simulink model "IEEE30_case"  (R2024b)
settings: Solver=FixedStepAuto  StartTime=0  StopTime=5  FixedStep=1e-7  RelTol=1e-3
values from neighbouring files (symbols this model uses):
  GFL_DFIG_7_C_bus = 0.08    [IEEE30_case_parameters.m]
  GFL_DFIG_7_D_mutual = 2.500000e+3    (= 2500)    [IEEE30_case_parameters.m]
  GFL_DFIG_7_f0 = 60    [IEEE30_case_parameters.m]
  GFL_DFIG_7_gPLLi = 3200    [IEEE30_case_parameters.m]
  GFL_DFIG_7_gPLLp = 650    [IEEE30_case_parameters.m]
  GFL_DFIG_7_H_WT = 0.4    [IEEE30_case_parameters.m]
  GFL_DFIG_7_Hg = 0.8    [IEEE30_case_parameters.m]
  GFL_DFIG_7_Igq_ref = 0    [IEEE30_case_parameters.m]
  GFL_DFIG_7_Ird_ref = 704.45696    [IEEE30_case_parameters.m]
  GFL_DFIG_7_KI_V = -300000    [IEEE30_case_parameters.m]
  GFL_DFIG_7_KP_V = -1000    [IEEE30_case_parameters.m]
  GFL_DFIG_7_Ksh = 1.254300e+4    (= 12543)    [IEEE30_case_parameters.m]
  GFL_DFIG_7_Lg = 0.000483    [IEEE30_case_parameters.m]
  GFL_DFIG_7_Lm_pu = 4    [IEEE30_case_parameters.m]
  GFL_DFIG_7_N = 100    [IEEE30_case_parameters.m]
  GFL_DFIG_7_p = 2    [IEEE30_case_parameters.m]
  GFL_DFIG_7_Pitch = 0    [IEEE30_case_parameters.m]
  GFL_DFIG_7_R = 44    [IEEE30_case_parameters.m]
  GFL_DFIG_7_Rg = 2.000000e-5    (= 2e-05)    [IEEE30_case_parameters.m]
  GFL_DFIG_7_rho = 1.225    [IEEE30_case_parameters.m]
  GFL_DFIG_7_rPLLi = 4500    [IEEE30_case_parameters.m]
  GFL_DFIG_7_rPLLp = 620    [IEEE30_case_parameters.m]
  GFL_DFIG_7_Rs_pu = 0.011    [IEEE30_case_parameters.m]
  GFL_DFIG_7_Sbase = 2.000000e+6    (= 2000000)    [IEEE30_case_parameters.m]
  GFL_DFIG_7_ugq_ref = 0    [IEEE30_case_parameters.m]
  GFL_DFIG_7_usd_ref = 0    [IEEE30_case_parameters.m]
  GFL_DFIG_7_Vbase = 690    [IEEE30_case_parameters.m]
  GFL_DFIG_7_Vdc_ref = 1200    [IEEE30_case_parameters.m]
  GFL_DFIG_7_wind = 12    [IEEE30_case_parameters.m]
  GFL_DFIG_7_wm_ref = 518.184209    [IEEE30_case_parameters.m]
  SG_D_13_D = 0.01056    [IEEE30_case_parameters.m]
  SG_D_13_EnableSaturation = 0    [IEEE30_case_parameters.m]
  SG_D_13_f0 = 60    [IEEE30_case_parameters.m]
  SG_D_13_H = 7.5    [IEEE30_case_parameters.m]
  SG_D_13_K_A = 20    [IEEE30_case_parameters.m]
  SG_D_13_K_E = 1.000000e+1    (= 10)    [IEEE30_case_parameters.m]
  SG_D_13_K_F = 2.363    [IEEE30_case_parameters.m]
  SG_D_13_K_s = 0.5    [IEEE30_case_parameters.m]
  SG_D_13_R_a = 0.001088    [IEEE30_case_parameters.m]
  SG_D_13_S_A = 1    [IEEE30_case_parameters.m]
  SG_D_13_S_B = 0.103    [IEEE30_case_parameters.m]
  SG_D_13_S_N = 10.659857    [IEEE30_case_parameters.m]
  SG_D_13_SpeedPara = 200    [IEEE30_case_parameters.m]
  SG_D_13_T_0 = 0.370163    [IEEE30_case_parameters.m]
  SG_D_13_T_1 = 0.3    [IEEE30_case_parameters.m]
  SG_D_13_T_2 = 0.05    [IEEE30_case_parameters.m]
  SG_D_13_T_3 = 0.02    [IEEE30_case_parameters.m]
  SG_D_13_T_4 = 0.005    [IEEE30_case_parameters.m]
  SG_D_13_T_A = 0.02    [IEEE30_case_parameters.m]
  SG_D_13_T_dd = 8.000000e+0    (= 8)    [IEEE30_case_parameters.m]
  SG_D_13_T_ddd = 0.04    [IEEE30_case_parameters.m]
  SG_D_13_T_E = 0.314    [IEEE30_case_parameters.m]
  SG_D_13_T_F = 0.35    [IEEE30_case_parameters.m]
  SG_D_13_T_qd = 0.8    [IEEE30_case_parameters.m]
  SG_D_13_T_qdd = 0.02    [IEEE30_case_parameters.m]
  SG_D_13_T_speed = 0.1    [IEEE30_case_parameters.m]
  SG_D_13_T_w = 0.5    [IEEE30_case_parameters.m]
  SG_D_13_V_ref = 1.696619    [IEEE30_case_parameters.m]
  SG_D_13_w_ref = 376.991118    [IEEE30_case_parameters.m]
  SG_D_13_x_d = 1.9    [IEEE30_case_parameters.m]
  SG_D_13_x_dd = 0.302    [IEEE30_case_parameters.m]
  SG_D_13_x_ddd = 0.204    [IEEE30_case_parameters.m]
  SG_D_13_x_l = 0.05    [IEEE30_case_parameters.m]
  SG_D_13_x_q = 1.3    [IEEE30_case_parameters.m]
  SG_D_13_x_qd = 0.5    [IEEE30_case_parameters.m]
  SG_D_13_x_qdd = 0.3    [IEEE30_case_parameters.m]
  SG_D_1_D = 0.01056    [IEEE30_case_parameters.m]
  SG_D_1_EnableSaturation = 0    [IEEE30_case_parameters.m]
  SG_D_1_f0 = 60    [IEEE30_case_parameters.m]
  SG_D_1_H = 7.5    [IEEE30_case_parameters.m]
  SG_D_1_K_A = 20    [IEEE30_case_parameters.m]
  SG_D_1_K_E = 1.000000e+1    (= 10)    [IEEE30_case_parameters.m]
  SG_D_1_K_F = 2.363    [IEEE30_case_parameters.m]
  SG_D_1_K_s = 0.5    [IEEE30_case_parameters.m]
  SG_D_1_R_a = 0.001088    [IEEE30_case_parameters.m]
  SG_D_1_S_A = 1    [IEEE30_case_parameters.m]
  SG_D_1_S_B = 0.103    [IEEE30_case_parameters.m]
  SG_D_1_S_N = 10.659857    [IEEE30_case_parameters.m]
  SG_D_1_SpeedPara = 200    [IEEE30_case_parameters.m]
  SG_D_1_T_0 = 0.259812    [IEEE30_case_parameters.m]
  SG_D_1_T_1 = 0.3    [IEEE30_case_parameters.m]
  SG_D_1_T_2 = 0.05    [IEEE30_case_parameters.m]
  SG_D_1_T_3 = 0.02    [IEEE30_case_parameters.m]
  SG_D_1_T_4 = 0.005    [IEEE30_case_parameters.m]
  SG_D_1_T_A = 0.02    [IEEE30_case_parameters.m]
  SG_D_1_T_dd = 8.000000e+0    (= 8)    [IEEE30_case_parameters.m]
  SG_D_1_T_ddd = 0.04    [IEEE30_case_parameters.m]
  SG_D_1_T_E = 0.314    [IEEE30_case_parameters.m]
  SG_D_1_T_F = 0.35    [IEEE30_case_parameters.m]
  SG_D_1_T_qd = 0.8    [IEEE30_case_parameters.m]
  SG_D_1_T_qdd = 0.02    [IEEE30_case_parameters.m]
  SG_D_1_T_speed = 0.1    [IEEE30_case_parameters.m]
  SG_D_1_T_w = 0.5    [IEEE30_case_parameters.m]
  SG_D_1_V_ref = 1.544107    [IEEE30_case_parameters.m]
  SG_D_1_w_ref = 376.991118    [IEEE30_case_parameters.m]
  SG_D_1_x_d = 1.9    [IEEE30_case_parameters.m]
  SG_D_1_x_dd = 0.302    [IEEE30_case_parameters.m]
  SG_D_1_x_ddd = 0.204    [IEEE30_case_parameters.m]
  SG_D_1_x_l = 0.05    [IEEE30_case_parameters.m]
  SG_D_1_x_q = 1.3    [IEEE30_case_parameters.m]
  SG_D_1_x_qd = 0.5    [IEEE30_case_parameters.m]
  SG_D_1_x_qdd = 0.3    [IEEE30_case_parameters.m]
  SG_D_22_D = 0.01056    [IEEE30_case_parameters.m]
  SG_D_22_EnableSaturation = 0    [IEEE30_case_parameters.m]
  SG_D_22_f0 = 60    [IEEE30_case_parameters.m]
  SG_D_22_H = 7.5    [IEEE30_case_parameters.m]
  SG_D_22_K_A = 20    [IEEE30_case_parameters.m]
  SG_D_22_K_E = 1.000000e+1    (= 10)    [IEEE30_case_parameters.m]
  SG_D_22_K_F = 2.363    [IEEE30_case_parameters.m]
  SG_D_22_K_s = 0.5    [IEEE30_case_parameters.m]
  SG_D_22_R_a = 0.001088    [IEEE30_case_parameters.m]
  SG_D_22_S_A = 1    [IEEE30_case_parameters.m]
  SG_D_22_S_B = 0.103    [IEEE30_case_parameters.m]
  SG_D_22_S_N = 10.659857    [IEEE30_case_parameters.m]
  SG_D_22_SpeedPara = 200    [IEEE30_case_parameters.m]
  SG_D_22_T_0 = 0.216121    [IEEE30_case_parameters.m]
  SG_D_22_T_1 = 0.3    [IEEE30_case_parameters.m]
  SG_D_22_T_2 = 0.05    [IEEE30_case_parameters.m]
  SG_D_22_T_3 = 0.02    [IEEE30_case_parameters.m]
  SG_D_22_T_4 = 0.005    [IEEE30_case_parameters.m]
  ... (+126 more)
(part 7 of 27)

== system IEEE30_case/AC_1/d_iq_line_10_21_block ==
  note: d_iq_line_10_21 in IEEE30_case
      | $5385.58740615393\,\mathrm{vq}_{\mathrm{bus},10}-161.567622184618\,\mathrm{iq}_{\mathrm{line},10,21}-376.991118430775\,\mathrm{id}_{\mathrm{line},10,21}-5385.58740615393\,\mathrm{vq}_{\mathrm{bus},21}$
      | Automatically generated on 2025-11-01 18:41:58 .
  State_id_line_10_21_eaa10 : Inport
  State_iq_line_10_21_3e3dc : Inport  Port=2
  State_vq_bus_10_d2e20 : Inport  Port=3
  State_vq_bus_21_091f2 : Inport  Port=4
  Add_26c65 : Sum
  Constant_-376.991118430775_c6985 : Constant  Value=-376.991118430775
  Constant_161.567622184618_102ba : Constant  Value=161.567622184618
  Constant_5385.58740615393_07e60 : Constant  Value=5385.58740615393
  Constant_5385.58740615393_39994 : Constant  Value=5385.58740615393
  Product_149d6 : Product
  Product_44b69 : Product
  Product_4a08d : Product
  Product_e31d5 : Product
  Subtract_26c55 : Sum  Inputs=+-
  Subtract_2b805 : Sum  Inputs=+-
  Blockout_d_iq_line_10_21_9f8c0 : Outport
  wires:
  Constant_-376.991118430775_c6985/1 -> Product_44b69/1
  Product_44b69/1 -> Subtract_2b805/1
  State_id_line_10_21_eaa10/1 -> Product_44b69/2
  Constant_161.567622184618_102ba/1 -> Product_149d6/1
  State_iq_line_10_21_3e3dc/1 -> Product_149d6/2
  Product_149d6/1 -> Subtract_2b805/2
  State_vq_bus_10_d2e20/1 -> Product_e31d5/2
  Product_e31d5/1 -> Add_26c65/2
  Constant_5385.58740615393_07e60/1 -> Product_e31d5/1
  Subtract_2b805/1 -> Add_26c65/1
  Product_4a08d/1 -> Subtract_26c55/2
  Constant_5385.58740615393_39994/1 -> Product_4a08d/1
  State_vq_bus_21_091f2/1 -> Product_4a08d/2
  Add_26c65/1 -> Subtract_26c55/1
  Subtract_26c55/1 -> Blockout_d_iq_line_10_21_9f8c0/1

== system IEEE30_case/AC_1/d_iq_line_10_22_block ==
  note: d_iq_line_10_22 in IEEE30_case
      | $2513.27412287183\,\mathrm{vq}_{\mathrm{bus},10}-175.929188601028\,\mathrm{iq}_{\mathrm{line},10,22}-376.991118430775\,\mathrm{id}_{\mathrm{line},10,22}-2513.27412287183\,\mathrm{vq}_{\mathrm{bus},22}$
      | Automatically generated on 2025-11-01 18:42:00 .
  State_id_line_10_22_084f6 : Inport
  State_iq_line_10_22_3080a : Inport  Port=2
  State_vq_bus_10_6b45e : Inport  Port=3
  State_vq_bus_22_cc06f : Inport  Port=4
  Add_09135 : Sum
  Constant_-376.991118430775_75af6 : Constant  Value=-376.991118430775
  Constant_175.929188601028_09936 : Constant  Value=175.929188601028
  Constant_2513.27412287183_cbdf1 : Constant  Value=2513.27412287183
  Constant_2513.27412287183_d3008 : Constant  Value=2513.27412287183
  Product_19b88 : Product
  Product_591c9 : Product
  Product_bc67e : Product
  Product_ee7ea : Product
  Subtract_086ed : Sum  Inputs=+-
  Subtract_aa73f : Sum  Inputs=+-
  Blockout_d_iq_line_10_22_034e5 : Outport
  wires:
  Constant_-376.991118430775_75af6/1 -> Product_ee7ea/1
  State_id_line_10_22_084f6/1 -> Product_ee7ea/2
  Constant_175.929188601028_09936/1 -> Product_19b88/1
  Product_19b88/1 -> Subtract_aa73f/2
  Product_591c9/1 -> Add_09135/2
  Constant_2513.27412287183_cbdf1/1 -> Product_591c9/1
  State_iq_line_10_22_3080a/1 -> Product_19b88/2
  Product_ee7ea/1 -> Subtract_aa73f/1
  State_vq_bus_10_6b45e/1 -> Product_591c9/2
  Subtract_aa73f/1 -> Add_09135/1
  Product_bc67e/1 -> Subtract_086ed/2
  Constant_2513.27412287183_d3008/1 -> Product_bc67e/1
  State_vq_bus_22_cc06f/1 -> Product_bc67e/2
  Add_09135/1 -> Subtract_086ed/1
  Subtract_086ed/1 -> Blockout_d_iq_line_10_22_034e5/1

== system IEEE30_case/AC_1/d_iq_line_12_13_block ==
  note: d_iq_line_12_13 in IEEE30_case
      | $2692.79370307697\,\mathrm{vq}_{\mathrm{bus},12}-376.991118430775\,\mathrm{id}_{\mathrm{line},12,13}-2692.79370307697\,\mathrm{vq}_{\mathrm{bus},13}$
      | Automatically generated on 2025-11-01 18:41:32 .
  State_id_line_12_13_e0b57 : Inport
  State_vq_bus_12_22143 : Inport  Port=2
  State_vq_bus_13_c3943 : Inport  Port=3
  Add_03ba8 : Sum
  Constant_-376.991118430775_53004 : Constant  Value=-376.991118430775
  Constant_2692.79370307697_acbc8 : Constant  Value=2692.79370307697
  Constant_2692.79370307697_b6261 : Constant  Value=2692.79370307697
  Product_60502 : Product
  Product_6a791 : Product
  Product_984e4 : Product
  Subtract_25f30 : Sum  Inputs=+-
  Blockout_d_iq_line_12_13_55f5a : Outport
  wires:
  Constant_-376.991118430775_53004/1 -> Product_6a791/1
  Constant_2692.79370307697_acbc8/1 -> Product_984e4/1
  Product_984e4/1 -> Add_03ba8/2
  Product_6a791/1 -> Add_03ba8/1
  State_id_line_12_13_e0b57/1 -> Product_6a791/2
  Product_60502/1 -> Subtract_25f30/2
  Constant_2692.79370307697_b6261/1 -> Product_60502/1
  State_vq_bus_12_22143/1 -> Product_984e4/2
  State_vq_bus_13_c3943/1 -> Product_60502/2
  Add_03ba8/1 -> Subtract_25f30/1
  Subtract_25f30/1 -> Blockout_d_iq_line_12_13_55f5a/1

== system IEEE30_case/AC_1/d_iq_line_12_14_block ==
  note: d_iq_line_12_14 in IEEE30_case
      | $1449.96584011837\,\mathrm{vq}_{\mathrm{bus},12}-173.995900814204\,\mathrm{iq}_{\mathrm{line},12,14}-376.991118430775\,\mathrm{id}_{\mathrm{line},12,14}-1449.96584011837\,\mathrm{vq}_{\mathrm{bus},14}$
      | Automatically generated on 2025-11-01 18:41:34 .
  State_id_line_12_14_b6e48 : Inport
  State_iq_line_12_14_89ecd : Inport  Port=2
  State_vq_bus_12_dcaec : Inport  Port=3
  State_vq_bus_14_44cc5 : Inport  Port=4
  Add_8fe1c : Sum
  Constant_-376.991118430775_6f91c : Constant  Value=-376.991118430775
  Constant_1449.96584011837_34179 : Constant  Value=1449.96584011837
  Constant_1449.96584011837_b6100 : Constant  Value=1449.96584011837
  Constant_173.995900814204_1440a : Constant  Value=173.995900814204
  Product_07a6c : Product
  Product_0c37e : Product
  Product_14585 : Product
  Product_d0fc4 : Product
  Subtract_a883b : Sum  Inputs=+-
  Subtract_dbef5 : Sum  Inputs=+-
  Blockout_d_iq_line_12_14_a9efb : Outport
  wires:
  State_iq_line_12_14_89ecd/1 -> Product_07a6c/2
  Constant_-376.991118430775_6f91c/1 -> Product_d0fc4/1
  Constant_173.995900814204_1440a/1 -> Product_07a6c/1
  Product_07a6c/1 -> Subtract_dbef5/2
  State_id_line_12_14_b6e48/1 -> Product_d0fc4/2
  Product_d0fc4/1 -> Subtract_dbef5/1
  Constant_1449.96584011837_b6100/1 -> Product_0c37e/1
  State_vq_bus_12_dcaec/1 -> Product_0c37e/2
  Subtract_dbef5/1 -> Add_8fe1c/1
  Product_0c37e/1 -> Add_8fe1c/2
  Product_14585/1 -> Subtract_a883b/2
  Constant_1449.96584011837_34179/1 -> Product_14585/1
  State_vq_bus_14_44cc5/1 -> Product_14585/2
  Add_8fe1c/1 -> Subtract_a883b/1
  Subtract_a883b/1 -> Blockout_d_iq_line_12_14_a9efb/1

== system IEEE30_case/AC_1/d_iq_line_12_15_block ==
  note: d_iq_line_12_15 in IEEE30_case
      | $2899.93168023673\,\mathrm{vq}_{\mathrm{bus},12}-202.995217616571\,\mathrm{iq}_{\mathrm{line},12,15}-376.991118430775\,\mathrm{id}_{\mathrm{line},12,15}-2899.93168023673\,\mathrm{vq}_{\mathrm{bus},15}$
      | Automatically generated on 2025-11-01 18:41:37 .
  State_id_line_12_15_beed2 : Inport
  State_iq_line_12_15_4b1af : Inport  Port=2
  State_vq_bus_12_5723c : Inport  Port=3
  State_vq_bus_15_811f3 : Inport  Port=4
  Add_8ef8f : Sum
  Constant_-376.991118430775_4e1e9 : Constant  Value=-376.991118430775
  Constant_202.995217616571_fe4cc : Constant  Value=202.995217616571
  Constant_2899.93168023673_6dafa : Constant  Value=2899.93168023673
  Constant_2899.93168023673_db74e : Constant  Value=2899.93168023673
  Product_1019c : Product
  Product_410ea : Product
  Product_7c07b : Product
  Product_c4a2c : Product
  Subtract_52a59 : Sum  Inputs=+-
  Subtract_a4dad : Sum  Inputs=+-
  Blockout_d_iq_line_12_15_872fa : Outport
  wires:
  Constant_-376.991118430775_4e1e9/1 -> Product_1019c/1
  Product_1019c/1 -> Subtract_52a59/1
  State_id_line_12_15_beed2/1 -> Product_1019c/2
  Constant_202.995217616571_fe4cc/1 -> Product_410ea/1
  Product_410ea/1 -> Subtract_52a59/2
  State_iq_line_12_15_4b1af/1 -> Product_410ea/2
  Product_7c07b/1 -> Add_8ef8f/2
  Constant_2899.93168023673_6dafa/1 -> Product_7c07b/1
  State_vq_bus_12_5723c/1 -> Product_7c07b/2
  Subtract_52a59/1 -> Add_8ef8f/1
  Constant_2899.93168023673_db74e/1 -> Product_c4a2c/1
  State_vq_bus_15_811f3/1 -> Product_c4a2c/2
  Add_8ef8f/1 -> Subtract_a4dad/1
  Product_c4a2c/1 -> Subtract_a4dad/2
  Subtract_a4dad/1 -> Blockout_d_iq_line_12_15_872fa/1

== system IEEE30_case/AC_1/d_iq_line_12_16_block ==
  note: d_iq_line_12_16 in IEEE30_case
      | $1884.95559215388\,\mathrm{vq}_{\mathrm{bus},12}-169.646003293849\,\mathrm{iq}_{\mathrm{line},12,16}-376.991118430775\,\mathrm{id}_{\mathrm{line},12,16}-1884.95559215388\,\mathrm{vq}_{\mathrm{bus},16}$
      | Automatically generated on 2025-11-01 18:41:39 .
  State_id_line_12_16_32f87 : Inport
  State_iq_line_12_16_057ef : Inport  Port=2
  State_vq_bus_12_19670 : Inport  Port=3
  State_vq_bus_16_185e6 : Inport  Port=4
  Add_44e5e : Sum
  Constant_-376.991118430775_e69c0 : Constant  Value=-376.991118430775
  Constant_169.646003293849_5d481 : Constant  Value=169.646003293849
  Constant_1884.95559215388_470b5 : Constant  Value=1884.95559215388
  Constant_1884.95559215388_79483 : Constant  Value=1884.95559215388
  Product_1478d : Product
  Product_64d0b : Product
  Product_809b3 : Product
  Product_e344e : Product
  Subtract_a6d27 : Sum  Inputs=+-
  Subtract_c23ff : Sum  Inputs=+-
  Blockout_d_iq_line_12_16_07cfb : Outport
  wires:
  Constant_-376.991118430775_e69c0/1 -> Product_64d0b/1
  Product_e344e/1 -> Subtract_c23ff/2
  Product_64d0b/1 -> Subtract_c23ff/1
  State_id_line_12_16_32f87/1 -> Product_64d0b/2
  Constant_169.646003293849_5d481/1 -> Product_e344e/1
  Product_809b3/1 -> Add_44e5e/2
  Constant_1884.95559215388_470b5/1 -> Product_809b3/1
  State_iq_line_12_16_057ef/1 -> Product_e344e/2
  State_vq_bus_12_19670/1 -> Product_809b3/2
  Subtract_c23ff/1 -> Add_44e5e/1
  Product_1478d/1 -> Subtract_a6d27/2
  Constant_1884.95559215388_79483/1 -> Product_1478d/1
  State_vq_bus_16_185e6/1 -> Product_1478d/2
  Add_44e5e/1 -> Subtract_a6d27/1
  Subtract_a6d27/1 -> Blockout_d_iq_line_12_16_07cfb/1

== system IEEE30_case/AC_1/d_iq_line_14_15_block ==
  note: d_iq_line_14_15 in IEEE30_case
      | $1884.95559215388\,\mathrm{vq}_{\mathrm{bus},14}-414.690230273853\,\mathrm{iq}_{\mathrm{line},14,15}-376.991118430775\,\mathrm{id}_{\mathrm{line},14,15}-1884.95559215388\,\mathrm{vq}_{\mathrm{bus},15}$
      | Automatically generated on 2025-11-01 18:41:42 .
  State_id_line_14_15_7494d : Inport
  State_iq_line_14_15_6bca3 : Inport  Port=2
  State_vq_bus_14_61922 : Inport  Port=3
  State_vq_bus_15_80bf7 : Inport  Port=4
  Add_1b324 : Sum
  Constant_-376.991118430775_071d9 : Constant  Value=-376.991118430775
  Constant_1884.95559215388_19c19 : Constant  Value=1884.95559215388
  Constant_1884.95559215388_3b58e : Constant  Value=1884.95559215388
  Constant_414.690230273853_bfc7a : Constant  Value=414.690230273853
  Product_525e6 : Product
  Product_5c681 : Product
  Product_e29bf : Product
  Product_e4297 : Product
  Subtract_00799 : Sum  Inputs=+-
  Subtract_f1741 : Sum  Inputs=+-
  Blockout_d_iq_line_14_15_23a62 : Outport
  wires:
  Constant_-376.991118430775_071d9/1 -> Product_e4297/1
  Constant_414.690230273853_bfc7a/1 -> Product_5c681/1
  Product_5c681/1 -> Subtract_00799/2
  State_id_line_14_15_7494d/1 -> Product_e4297/2
  State_iq_line_14_15_6bca3/1 -> Product_5c681/2
  Product_e4297/1 -> Subtract_00799/1
  State_vq_bus_14_61922/1 -> Product_525e6/2
  Product_525e6/1 -> Add_1b324/2
  Constant_1884.95559215388_3b58e/1 -> Product_525e6/1
  Subtract_00799/1 -> Add_1b324/1
  Product_e29bf/1 -> Subtract_f1741/2
  Constant_1884.95559215388_19c19/1 -> Product_e29bf/1
  Add_1b324/1 -> Subtract_f1741/1
  State_vq_bus_15_80bf7/1 -> Product_e29bf/2
  Subtract_f1741/1 -> Blockout_d_iq_line_14_15_23a62/1

== system IEEE30_case/AC_1/d_iq_line_15_18_block ==
  note: d_iq_line_15_18 in IEEE30_case
      | $1713.59599286716\,\mathrm{vq}_{\mathrm{bus},15}-188.495559215388\,\mathrm{iq}_{\mathrm{line},15,18}-376.991118430775\,\mathrm{id}_{\mathrm{line},15,18}-1713.59599286716\,\mathrm{vq}_{\mathrm{bus},18}$
      | Automatically generated on 2025-11-01 18:41:46 .
  State_id_line_15_18_c7b72 : Inport
  State_iq_line_15_18_85966 : Inport  Port=2
  State_vq_bus_15_ceac7 : Inport  Port=3
  State_vq_bus_18_6e5b1 : Inport  Port=4
  Add_a8775 : Sum
  Constant_-376.991118430775_1952d : Constant  Value=-376.991118430775
  Constant_1713.59599286716_867a5 : Constant  Value=1713.59599286716
  Constant_1713.59599286716_e050c : Constant  Value=1713.59599286716
  Constant_188.495559215388_7a49f : Constant  Value=188.495559215388
  Product_51a61 : Product
  Product_be0d8 : Product
  Product_ded70 : Product
  Product_e1c77 : Product
  Subtract_50270 : Sum  Inputs=+-
  Subtract_cf1ed : Sum  Inputs=+-
  Blockout_d_iq_line_15_18_9343c : Outport
  wires:
  Constant_-376.991118430775_1952d/1 -> Product_be0d8/1
  Constant_188.495559215388_7a49f/1 -> Product_e1c77/1
  Product_e1c77/1 -> Subtract_cf1ed/2
  Product_be0d8/1 -> Subtract_cf1ed/1
  State_id_line_15_18_c7b72/1 -> Product_be0d8/2
  Product_51a61/1 -> Add_a8775/2
  Constant_1713.59599286716_e050c/1 -> Product_51a61/1
  State_iq_line_15_18_85966/1 -> Product_e1c77/2
  State_vq_bus_15_ceac7/1 -> Product_51a61/2
  Subtract_cf1ed/1 -> Add_a8775/1
  Constant_1713.59599286716_867a5/1 -> Product_ded70/1
  State_vq_bus_18_6e5b1/1 -> Product_ded70/2
  Add_a8775/1 -> Subtract_50270/1
  Product_ded70/1 -> Subtract_50270/2
  Subtract_50270/1 -> Blockout_d_iq_line_15_18_9343c/1

== system IEEE30_case/AC_1/d_iq_line_15_23_block ==
  note: d_iq_line_15_23 in IEEE30_case
      | $1884.95559215388\,\mathrm{vq}_{\mathrm{bus},15}-188.495559215388\,\mathrm{iq}_{\mathrm{line},15,23}-376.991118430775\,\mathrm{id}_{\mathrm{line},15,23}-1884.95559215388\,\mathrm{vq}_{\mathrm{bus},23}$
      | Automatically generated on 2025-11-01 18:42:05 .
  State_id_line_15_23_e0160 : Inport
  State_iq_line_15_23_ade94 : Inport  Port=2
  State_vq_bus_15_76336 : Inport  Port=3
  State_vq_bus_23_32b73 : Inport  Port=4
  Add_e2306 : Sum
  Constant_-376.991118430775_e195e : Constant  Value=-376.991118430775
  Constant_188.495559215388_43fcb : Constant  Value=188.495559215388
  Constant_1884.95559215388_4e938 : Constant  Value=1884.95559215388
  Constant_1884.95559215388_b35ae : Constant  Value=1884.95559215388
  Product_00db3 : Product
  Product_516e5 : Product
  Product_90be9 : Product
  Product_b8377 : Product
  Subtract_711a0 : Sum  Inputs=+-
  Subtract_e6dfb : Sum  Inputs=+-
  Blockout_d_iq_line_15_23_620f2 : Outport
  wires:
  Constant_-376.991118430775_e195e/1 -> Product_90be9/1
  Product_90be9/1 -> Subtract_e6dfb/1
  Subtract_711a0/1 -> Blockout_d_iq_line_15_23_620f2/1
  State_id_line_15_23_e0160/1 -> Product_90be9/2
  Constant_188.495559215388_43fcb/1 -> Product_516e5/1
  Product_516e5/1 -> Subtract_e6dfb/2
  State_iq_line_15_23_ade94/1 -> Product_516e5/2
  Product_00db3/1 -> Add_e2306/2
  Constant_1884.95559215388_b35ae/1 -> Product_00db3/1
  State_vq_bus_15_76336/1 -> Product_00db3/2
  Subtract_e6dfb/1 -> Add_e2306/1
  Constant_1884.95559215388_4e938/1 -> Product_b8377/1
  State_vq_bus_23_32b73/1 -> Product_b8377/2
  Add_e2306/1 -> Subtract_711a0/1
  Product_b8377/1 -> Subtract_711a0/2

== system IEEE30_case/AC_1/d_iq_line_16_17_block ==
  note: d_iq_line_16_17 in IEEE30_case
      | $1984.16378121461\,\mathrm{vq}_{\mathrm{bus},16}-158.733102497168\,\mathrm{iq}_{\mathrm{line},16,17}-376.991118430775\,\mathrm{id}_{\mathrm{line},16,17}-1984.16378121461\,\mathrm{vq}_{\mathrm{bus},17}$
      | Automatically generated on 2025-11-01 18:41:44 .
  State_id_line_16_17_721a9 : Inport
  State_iq_line_16_17_c5f3c : Inport  Port=2
  State_vq_bus_16_312ae : Inport  Port=3
  State_vq_bus_17_5c6e8 : Inport  Port=4
  Add_ea472 : Sum
  Constant_-376.991118430775_937ec : Constant  Value=-376.991118430775
  Constant_158.733102497168_9c41c : Constant  Value=158.733102497168
  Constant_1984.16378121461_5691c : Constant  Value=1984.16378121461
  Constant_1984.16378121461_d1a9e : Constant  Value=1984.16378121461
  Product_1c0b5 : Product
  Product_32b71 : Product
  Product_382cd : Product
  Product_3fc5f : Product
  Subtract_3f09d : Sum  Inputs=+-
  Subtract_60968 : Sum  Inputs=+-
  Blockout_d_iq_line_16_17_36e2b : Outport
  wires:
  Product_1c0b5/1 -> Subtract_3f09d/1
  Constant_-376.991118430775_937ec/1 -> Product_1c0b5/1
  State_id_line_16_17_721a9/1 -> Product_1c0b5/2
  Constant_158.733102497168_9c41c/1 -> Product_3fc5f/1
  Product_3fc5f/1 -> Subtract_3f09d/2
  State_iq_line_16_17_c5f3c/1 -> Product_3fc5f/2
  Subtract_60968/1 -> Blockout_d_iq_line_16_17_36e2b/1
  Constant_1984.16378121461_5691c/1 -> Product_382cd/1
  State_vq_bus_16_312ae/1 -> Product_382cd/2
  Subtract_3f09d/1 -> Add_ea472/1
  Product_382cd/1 -> Add_ea472/2
  Product_32b71/1 -> Subtract_60968/2
  Constant_1984.16378121461_d1a9e/1 -> Product_32b71/1
  State_vq_bus_17_5c6e8/1 -> Product_32b71/2
  Add_ea472/1 -> Subtract_60968/1

== system IEEE30_case/AC_1/d_iq_line_18_19_block ==
  note: d_iq_line_18_19 in IEEE30_case
      | $2899.93168023673\,\mathrm{vq}_{\mathrm{bus},18}-173.995900814204\,\mathrm{iq}_{\mathrm{line},18,19}-376.991118430775\,\mathrm{id}_{\mathrm{line},18,19}-2899.93168023673\,\mathrm{vq}_{\mathrm{bus},19}$
      | Automatically generated on 2025-11-01 18:41:48 .
  State_id_line_18_19_8f9c3 : Inport
  State_iq_line_18_19_da0b4 : Inport  Port=2
  State_vq_bus_18_f4e53 : Inport  Port=3
  State_vq_bus_19_d8da0 : Inport  Port=4
  Add_013ce : Sum
  Constant_-376.991118430775_7eb58 : Constant  Value=-376.991118430775
  Constant_173.995900814204_e9e37 : Constant  Value=173.995900814204
  Constant_2899.93168023673_04a9c : Constant  Value=2899.93168023673
  Constant_2899.93168023673_0d6a4 : Constant  Value=2899.93168023673
  Product_2881c : Product
  Product_84c05 : Product
  Product_af8cd : Product
  Product_e9970 : Product
  Subtract_158eb : Sum  Inputs=+-
  Subtract_e49c7 : Sum  Inputs=+-
  Blockout_d_iq_line_18_19_0dac2 : Outport
  wires:
  Constant_-376.991118430775_7eb58/1 -> Product_e9970/1
  Product_e9970/1 -> Subtract_158eb/1
  State_id_line_18_19_8f9c3/1 -> Product_e9970/2
  Constant_173.995900814204_e9e37/1 -> Product_2881c/1
  Product_84c05/1 -> Add_013ce/2
  Constant_2899.93168023673_04a9c/1 -> Product_84c05/1
  State_iq_line_18_19_da0b4/1 -> Product_2881c/2
  State_vq_bus_18_f4e53/1 -> Product_84c05/2
  Product_2881c/1 -> Subtract_158eb/2
  Subtract_158eb/1 -> Add_013ce/1
  Product_af8cd/1 -> Subtract_e49c7/2
  Constant_2899.93168023673_0d6a4/1 -> Product_af8cd/1
  State_vq_bus_19_d8da0/1 -> Product_af8cd/2
  Add_013ce/1 -> Subtract_e49c7/1
  Subtract_e49c7/1 -> Blockout_d_iq_line_18_19_0dac2/1

== system IEEE30_case/AC_1/d_iq_line_19_20_block ==
  note: d_iq_line_19_20 in IEEE30_case
      | $5385.58740615393\,\mathrm{vq}_{\mathrm{bus},19}-161.567622184618\,\mathrm{iq}_{\mathrm{line},19,20}-376.991118430775\,\mathrm{id}_{\mathrm{line},19,20}-5385.58740615393\,\mathrm{vq}_{\mathrm{bus},20}$
      | Automatically generated on 2025-11-01 18:41:50 .
  State_id_line_19_20_b531a : Inport
  State_iq_line_19_20_2451d : Inport  Port=2
  State_vq_bus_19_a0dab : Inport  Port=3
  State_vq_bus_20_72c0e : Inport  Port=4
  Add_bef5a : Sum
  Constant_-376.991118430775_a4716 : Constant  Value=-376.991118430775
  Constant_161.567622184618_2b234 : Constant  Value=161.567622184618
  Constant_5385.58740615393_0368b : Constant  Value=5385.58740615393
  Constant_5385.58740615393_91113 : Constant  Value=5385.58740615393
  Product_5eee0 : Product
  Product_83d90 : Product
  Product_85c6d : Product
  Product_f88ed : Product
  Subtract_a0a7d : Sum  Inputs=+-
  Subtract_ee448 : Sum  Inputs=+-
  Blockout_d_iq_line_19_20_abe71 : Outport
  wires:
  Constant_-376.991118430775_a4716/1 -> Product_5eee0/1
  Constant_161.567622184618_2b234/1 -> Product_85c6d/1
  Product_85c6d/1 -> Subtract_a0a7d/2
  State_id_line_19_20_b531a/1 -> Product_5eee0/2
  State_iq_line_19_20_2451d/1 -> Product_85c6d/2
  Product_83d90/1 -> Add_bef5a/2
  Constant_5385.58740615393_0368b/1 -> Product_83d90/1
  Product_5eee0/1 -> Subtract_a0a7d/1
  State_vq_bus_19_a0dab/1 -> Product_83d90/2
  Subtract_a0a7d/1 -> Add_bef5a/1
  Product_f88ed/1 -> Subtract_ee448/2
  Constant_5385.58740615393_91113/1 -> Product_f88ed/1
  State_vq_bus_20_72c0e/1 -> Product_f88ed/2
  Add_bef5a/1 -> Subtract_ee448/1
  Subtract_ee448/1 -> Blockout_d_iq_line_19_20_abe71/1

== system IEEE30_case/AC_1/d_iq_line_1_2_block ==
  note: d_iq_line_1_2 in IEEE30_case
      | $6283.18530717959\,\mathrm{vq}_{\mathrm{bus},1}-125.663706143592\,\mathrm{iq}_{\mathrm{line},1,2}-376.991118430775\,\mathrm{id}_{\mathrm{line},1,2}-6283.18530717959\,\mathrm{vq}_{\mathrm{bus},2}$
      | Automatically generated on 2025-11-01 18:40:58 .
  State_id_line_1_2_bca8d : Inport
  State_iq_line_1_2_62f2c : Inport  Port=2
  State_vq_bus_1_1d692 : Inport  Port=3
  State_vq_bus_2_54dcd : Inport  Port=4
  Add_b2adf : Sum
  Constant_-376.991118430775_ca98e : Constant  Value=-376.991118430775
  Constant_125.663706143592_a8407 : Constant  Value=125.663706143592
  Constant_6283.18530717959_17d64 : Constant  Value=6283.18530717959
  Constant_6283.18530717959_801ca : Constant  Value=6283.18530717959
  Product_34205 : Product
  Product_a0ca5 : Product
  Product_dcbb8 : Product
  Product_df49a : Product
  Subtract_4031b : Sum  Inputs=+-
  Subtract_ffb91 : Sum  Inputs=+-
  Blockout_d_iq_line_1_2_85e11 : Outport
  wires:
  Constant_-376.991118430775_ca98e/1 -> Product_df49a/1
  Product_dcbb8/1 -> Subtract_4031b/2
  Constant_6283.18530717959_17d64/1 -> Product_dcbb8/1
  Product_df49a/1 -> Subtract_ffb91/1
  State_id_line_1_2_bca8d/1 -> Product_df49a/2
  Constant_125.663706143592_a8407/1 -> Product_a0ca5/1
  Product_34205/1 -> Add_b2adf/2
  State_iq_line_1_2_62f2c/1 -> Product_a0ca5/2
  Constant_6283.18530717959_801ca/1 -> Product_34205/1
  Product_a0ca5/1 -> Subtract_ffb91/2
  State_vq_bus_1_1d692/1 -> Product_34205/2
  Subtract_ffb91/1 -> Add_b2adf/1
  State_vq_bus_2_54dcd/1 -> Product_dcbb8/2
  Add_b2adf/1 -> Subtract_4031b/1
  Subtract_4031b/1 -> Blockout_d_iq_line_1_2_85e11/1

== system IEEE30_case/AC_1/d_iq_line_1_3_block ==
  note: d_iq_line_1_3 in IEEE30_case
      | $1984.16378121461\,\mathrm{vq}_{\mathrm{bus},1}-99.2081890607303\,\mathrm{iq}_{\mathrm{line},1,3}-376.991118430775\,\mathrm{id}_{\mathrm{line},1,3}-1984.16378121461\,\mathrm{vq}_{\mathrm{bus},3}$
      | Automatically generated on 2025-11-01 18:41:00 .
  State_id_line_1_3_ae183 : Inport
  State_iq_line_1_3_f4510 : Inport  Port=2
  State_vq_bus_1_564cd : Inport  Port=3
  State_vq_bus_3_23559 : Inport  Port=4
  Add_e4d90 : Sum
  Constant_-376.991118430775_b2df0 : Constant  Value=-376.991118430775
  Constant_1984.16378121461_0937d : Constant  Value=1984.16378121461
  Constant_1984.16378121461_24c35 : Constant  Value=1984.16378121461
  Constant_99.2081890607303_19836 : Constant  Value=99.2081890607303
  Product_19dbd : Product
  Product_63c3f : Product
  Product_dc168 : Product
  Product_f16ee : Product
  Subtract_53029 : Sum  Inputs=+-
  Subtract_82ef4 : Sum  Inputs=+-
  Blockout_d_iq_line_1_3_dab4a : Outport
  wires:
  Constant_-376.991118430775_b2df0/1 -> Product_63c3f/1
  State_id_line_1_3_ae183/1 -> Product_63c3f/2
  Constant_99.2081890607303_19836/1 -> Product_19dbd/1
  Product_19dbd/1 -> Subtract_53029/2
  State_iq_line_1_3_f4510/1 -> Product_19dbd/2
  Product_f16ee/1 -> Add_e4d90/2
  Product_63c3f/1 -> Subtract_53029/1
  Constant_1984.16378121461_0937d/1 -> Product_f16ee/1
  State_vq_bus_1_564cd/1 -> Product_f16ee/2
  Subtract_53029/1 -> Add_e4d90/1
  Product_dc168/1 -> Subtract_82ef4/2
  Constant_1984.16378121461_24c35/1 -> Product_dc168/1
  State_vq_bus_3_23559/1 -> Product_dc168/2
  Add_e4d90/1 -> Subtract_82ef4/1
  Subtract_82ef4/1 -> Blockout_d_iq_line_1_3_dab4a/1

== system IEEE30_case/AC_1/d_iq_line_21_22_block ==
  note: d_iq_line_21_22 in IEEE30_case
      | $18849.5559215388\,\mathrm{vq}_{\mathrm{bus},21}-188.495559215388\,\mathrm{iq}_{\mathrm{line},21,22}-376.991118430775\,\mathrm{id}_{\mathrm{line},21,22}-18849.5559215388\,\mathrm{vq}_{\mathrm{bus},22}$
      | Automatically generated on 2025-11-01 18:42:02 .
  State_id_line_21_22_6fd19 : Inport
  State_iq_line_21_22_2fa40 : Inport  Port=2
  State_vq_bus_21_8118e : Inport  Port=3
  State_vq_bus_22_8ed98 : Inport  Port=4
  Add_1c3f8 : Sum
  Constant_-376.991118430775_126f8 : Constant  Value=-376.991118430775
  Constant_188.495559215388_db26c : Constant  Value=188.495559215388
  Constant_18849.5559215388_0d0d0 : Constant  Value=18849.5559215388
  Constant_18849.5559215388_e3d62 : Constant  Value=18849.5559215388
  Product_03a6b : Product
  Product_08fdc : Product
  Product_209a0 : Product
  Product_6e1ba : Product
  Subtract_39b85 : Sum  Inputs=+-
  Subtract_e1a2e : Sum  Inputs=+-
  Blockout_d_iq_line_21_22_19dd1 : Outport
  wires:
  State_iq_line_21_22_2fa40/1 -> Product_6e1ba/2
  Constant_-376.991118430775_126f8/1 -> Product_03a6b/1
  Constant_188.495559215388_db26c/1 -> Product_6e1ba/1
  Product_6e1ba/1 -> Subtract_39b85/2
  State_id_line_21_22_6fd19/1 -> Product_03a6b/2
  Product_03a6b/1 -> Subtract_39b85/1
  Constant_18849.5559215388_e3d62/1 -> Product_08fdc/1
  State_vq_bus_21_8118e/1 -> Product_08fdc/2
  Subtract_39b85/1 -> Add_1c3f8/1
  Product_08fdc/1 -> Add_1c3f8/2
  Product_209a0/1 -> Subtract_e1a2e/2
  Constant_18849.5559215388_0d0d0/1 -> Product_209a0/1
  State_vq_bus_22_8ed98/1 -> Product_209a0/2
  Add_1c3f8/1 -> Subtract_e1a2e/1
  Subtract_e1a2e/1 -> Blockout_d_iq_line_21_22_19dd1/1

== system IEEE30_case/AC_1/d_iq_line_22_24_block ==
  note: d_iq_line_22_24 in IEEE30_case
      | $2094.39510239319\,\mathrm{vq}_{\mathrm{bus},22}-251.327412287183\,\mathrm{iq}_{\mathrm{line},22,24}-376.991118430775\,\mathrm{id}_{\mathrm{line},22,24}-2094.39510239319\,\mathrm{vq}_{\mathrm{bus},24}$
      | Automatically generated on 2025-11-01 18:42:07 .
  State_id_line_22_24_f3c92 : Inport
  State_iq_line_22_24_cd212 : Inport  Port=2
  State_vq_bus_22_11d1c : Inport  Port=3
  State_vq_bus_24_1befd : Inport  Port=4
  Add_4a08e : Sum
  Constant_-376.991118430775_c447d : Constant  Value=-376.991118430775
  Constant_2094.39510239319_b8498 : Constant  Value=2094.39510239319
  Constant_2094.39510239319_c9baf : Constant  Value=2094.39510239319
  Constant_251.327412287183_d3184 : Constant  Value=251.327412287183
  Product_1b188 : Product
  Product_37c41 : Product
  Product_66b2f : Product
  Product_ef712 : Product
  Subtract_2094f : Sum  Inputs=+-
  Subtract_4ab50 : Sum  Inputs=+-
  Blockout_d_iq_line_22_24_c0f91 : Outport
  wires:
  Constant_-376.991118430775_c447d/1 -> Product_66b2f/1
  Product_66b2f/1 -> Subtract_4ab50/1
  State_id_line_22_24_f3c92/1 -> Product_66b2f/2
  Constant_251.327412287183_d3184/1 -> Product_1b188/1
  Product_ef712/1 -> Add_4a08e/2
  Constant_2094.39510239319_b8498/1 -> Product_ef712/1
  State_iq_line_22_24_cd212/1 -> Product_1b188/2
  State_vq_bus_22_11d1c/1 -> Product_ef712/2
  Product_1b188/1 -> Subtract_4ab50/2
  Subtract_4ab50/1 -> Add_4a08e/1
  Product_37c41/1 -> Subtract_2094f/2
  Constant_2094.39510239319_c9baf/1 -> Product_37c41/1
  State_vq_bus_24_1befd/1 -> Product_37c41/2
  Add_4a08e/1 -> Subtract_2094f/1
  Subtract_2094f/1 -> Blockout_d_iq_line_22_24_c0f91/1

== system IEEE30_case/AC_1/d_iq_line_23_24_block ==
  note: d_iq_line_23_24 in IEEE30_case
      | $1396.26340159546\,\mathrm{vq}_{\mathrm{bus},23}-181.51424220741\,\mathrm{iq}_{\mathrm{line},23,24}-376.991118430775\,\mathrm{id}_{\mathrm{line},23,24}-1396.26340159546\,\mathrm{vq}_{\mathrm{bus},24}$
      | Automatically generated on 2025-11-01 18:42:10 .
  State_id_line_23_24_71134 : Inport
  State_iq_line_23_24_146a4 : Inport  Port=2
  State_vq_bus_23_d5a58 : Inport  Port=3
  State_vq_bus_24_00c5d : Inport  Port=4
  Add_f0d22 : Sum
  Constant_-376.991118430775_47d54 : Constant  Value=-376.991118430775
  Constant_1396.26340159546_6a6eb : Constant  Value=1396.26340159546
  Constant_1396.26340159546_dcfdb : Constant  Value=1396.26340159546
  Constant_181.51424220741_fe7cc : Constant  Value=181.51424220741
  Product_4a48d : Product
  Product_614e0 : Product
  Product_ac60b : Product
  Product_caaa2 : Product
  Subtract_cb232 : Sum  Inputs=+-
  Subtract_e8ce7 : Sum  Inputs=+-
  Blockout_d_iq_line_23_24_07ba5 : Outport
  wires:
  Constant_-376.991118430775_47d54/1 -> Product_614e0/1
  Constant_181.51424220741_fe7cc/1 -> Product_4a48d/1
  Product_4a48d/1 -> Subtract_e8ce7/2
  State_id_line_23_24_71134/1 -> Product_614e0/2
  State_iq_line_23_24_146a4/1 -> Product_4a48d/2
  Product_ac60b/1 -> Add_f0d22/2
  Constant_1396.26340159546_dcfdb/1 -> Product_ac60b/1
  Product_614e0/1 -> Subtract_e8ce7/1
  State_vq_bus_23_d5a58/1 -> Product_ac60b/2
  Subtract_e8ce7/1 -> Add_f0d22/1
  Product_caaa2/1 -> Subtract_cb232/2
  Constant_1396.26340159546_6a6eb/1 -> Product_caaa2/1
  State_vq_bus_24_00c5d/1 -> Product_caaa2/2
  Add_f0d22/1 -> Subtract_cb232/1
  Subtract_cb232/1 -> Blockout_d_iq_line_23_24_07ba5/1

== system IEEE30_case/AC_1/d_iq_line_24_25_block ==
  note: d_iq_line_24_25 in IEEE30_case
      | $1142.39732857811\,\mathrm{vq}_{\mathrm{bus},24}-217.05549242984\,\mathrm{iq}_{\mathrm{line},24,25}-376.991118430775\,\mathrm{id}_{\mathrm{line},24,25}-1142.39732857811\,\mathrm{vq}_{\mathrm{bus},25}$
      | Automatically generated on 2025-11-01 18:42:12 .
  State_id_line_24_25_c259a : Inport
  State_iq_line_24_25_774ec : Inport  Port=2
  State_vq_bus_24_1bac9 : Inport  Port=3
  State_vq_bus_25_584b4 : Inport  Port=4
  Add_f6098 : Sum
  Constant_-376.991118430775_500c0 : Constant  Value=-376.991118430775
  Constant_1142.39732857811_1ac9b : Constant  Value=1142.39732857811
  Constant_1142.39732857811_bb189 : Constant  Value=1142.39732857811
  Constant_217.05549242984_109cc : Constant  Value=217.05549242984
  Product_1ea6a : Product
  Product_6196c : Product
  Product_d39d4 : Product
  Product_ffbc3 : Product
  Subtract_3189a : Sum  Inputs=+-
  Subtract_40dce : Sum  Inputs=+-
  Blockout_d_iq_line_24_25_5a1b9 : Outport
  wires:
  Product_d39d4/1 -> Subtract_3189a/1
  Constant_-376.991118430775_500c0/1 -> Product_d39d4/1
  Subtract_40dce/1 -> Blockout_d_iq_line_24_25_5a1b9/1
  State_id_line_24_25_c259a/1 -> Product_d39d4/2
  Constant_217.05549242984_109cc/1 -> Product_1ea6a/1
  Product_1ea6a/1 -> Subtract_3189a/2
  State_iq_line_24_25_774ec/1 -> Product_1ea6a/2
  Constant_1142.39732857811_bb189/1 -> Product_ffbc3/1
  State_vq_bus_24_1bac9/1 -> Product_ffbc3/2
  Subtract_3189a/1 -> Add_f6098/1
  Product_ffbc3/1 -> Add_f6098/2
  Product_6196c/1 -> Subtract_40dce/2
  Constant_1142.39732857811_1ac9b/1 -> Product_6196c/1
  State_vq_bus_25_584b4/1 -> Product_6196c/2
  Add_f6098/1 -> Subtract_40dce/1

== system IEEE30_case/AC_1/d_iq_line_25_26_block ==
  note: d_iq_line_25_26 in IEEE30_case
      | $992.081890607303\,\mathrm{vq}_{\mathrm{bus},25}-248.020472651826\,\mathrm{iq}_{\mathrm{line},25,26}-376.991118430775\,\mathrm{id}_{\mathrm{line},25,26}-992.081890607303\,\mathrm{vq}_{\mathrm{bus},26}$
      | Automatically generated on 2025-11-01 18:42:14 .
  State_id_line_25_26_499e6 : Inport
  State_iq_line_25_26_5031e : Inport  Port=2
  State_vq_bus_25_a69b5 : Inport  Port=3
  State_vq_bus_26_76074 : Inport  Port=4
  Add_0b2c6 : Sum
  Constant_-376.991118430775_73e90 : Constant  Value=-376.991118430775
  Constant_248.020472651826_63ba9 : Constant  Value=248.020472651826
  Constant_992.081890607303_603f1 : Constant  Value=992.081890607303
  Constant_992.081890607303_89fb8 : Constant  Value=992.081890607303
  Product_2d696 : Product
  Product_b5193 : Product
  Product_bb719 : Product
  Product_ce612 : Product
  Subtract_2e74f : Sum  Inputs=+-
  Subtract_a14e5 : Sum  Inputs=+-
  Blockout_d_iq_line_25_26_d7e2d : Outport
  wires:
  Constant_-376.991118430775_73e90/1 -> Product_b5193/1
  Product_ce612/1 -> Add_0b2c6/2
  Constant_992.081890607303_89fb8/1 -> Product_ce612/1
  Product_b5193/1 -> Subtract_a14e5/1
  State_id_line_25_26_499e6/1 -> Product_b5193/2
  Constant_248.020472651826_63ba9/1 -> Product_bb719/1
  Product_bb719/1 -> Subtract_a14e5/2
  Subtract_2e74f/1 -> Blockout_d_iq_line_25_26_d7e2d/1
  State_iq_line_25_26_5031e/1 -> Product_bb719/2
  State_vq_bus_25_a69b5/1 -> Product_ce612/2
  Subtract_a14e5/1 -> Add_0b2c6/1
  Constant_992.081890607303_603f1/1 -> Product_2d696/1
  State_vq_bus_26_76074/1 -> Product_2d696/2
  Add_0b2c6/1 -> Subtract_2e74f/1
  Product_2d696/1 -> Subtract_2e74f/2

== system IEEE30_case/AC_1/d_iq_line_25_27_block ==
  note: d_iq_line_25_27 in IEEE30_case
      | $1795.19580205131\,\mathrm{vq}_{\mathrm{bus},25}-197.471538225644\,\mathrm{iq}_{\mathrm{line},25,27}-376.991118430775\,\mathrm{id}_{\mathrm{line},25,27}-1795.19580205131\,\mathrm{vq}_{\mathrm{bus},27}$
      | Automatically generated on 2025-11-01 18:42:17 .
  State_id_line_25_27_adc44 : Inport
  State_iq_line_25_27_e5d71 : Inport  Port=2
  State_vq_bus_25_cd5c7 : Inport  Port=3
  State_vq_bus_27_3c154 : Inport  Port=4
  Add_c370e : Sum
  Constant_-376.991118430775_d1caf : Constant  Value=-376.991118430775
  Constant_1795.19580205131_4df5b : Constant  Value=1795.19580205131
  Constant_1795.19580205131_e4e3b : Constant  Value=1795.19580205131
  Constant_197.471538225644_e3937 : Constant  Value=197.471538225644
  Product_1d6a8 : Product
  Product_270ef : Product
  Product_5a9c6 : Product
  Product_f49b7 : Product
  Subtract_6e796 : Sum  Inputs=+-
  Subtract_f11f9 : Sum  Inputs=+-
  Blockout_d_iq_line_25_27_06e15 : Outport
  wires:
  Constant_-376.991118430775_d1caf/1 -> Product_270ef/1
  Product_270ef/1 -> Subtract_6e796/1
  State_id_line_25_27_adc44/1 -> Product_270ef/2
  Subtract_6e796/1 -> Add_c370e/1
  Constant_197.471538225644_e3937/1 -> Product_f49b7/1
  State_iq_line_25_27_e5d71/1 -> Product_f49b7/2
  Product_f49b7/1 -> Subtract_6e796/2
  State_vq_bus_25_cd5c7/1 -> Product_5a9c6/2
  Product_5a9c6/1 -> Add_c370e/2
  Constant_1795.19580205131_4df5b/1 -> Product_5a9c6/1
  Product_1d6a8/1 -> Subtract_f11f9/2
  Constant_1795.19580205131_e4e3b/1 -> Product_1d6a8/1
  State_vq_bus_27_3c154/1 -> Product_1d6a8/2
  Add_c370e/1 -> Subtract_f11f9/1
  Subtract_f11f9/1 -> Blockout_d_iq_line_25_27_06e15/1

== system IEEE30_case/AC_1/d_iq_line_27_29_block ==
  note: d_iq_line_27_29 in IEEE30_case
      | $897.597901025655\,\mathrm{vq}_{\mathrm{bus},27}-197.471538225644\,\mathrm{iq}_{\mathrm{line},27,29}-376.991118430775\,\mathrm{id}_{\mathrm{line},27,29}-897.597901025655\,\mathrm{vq}_{\mathrm{bus},29}$
      | Automatically generated on 2025-11-01 18:42:21 .
  State_id_line_27_29_86314 : Inport
  State_iq_line_27_29_e2b12 : Inport  Port=2
  State_vq_bus_27_cc3b8 : Inport  Port=3
  State_vq_bus_29_394c9 : Inport  Port=4
  Add_01c7b : Sum
  Constant_-376.991118430775_e3c81 : Constant  Value=-376.991118430775
  Constant_197.471538225644_20461 : Constant  Value=197.471538225644
  Constant_897.597901025655_51739 : Constant  Value=897.597901025655
  Constant_897.597901025655_7ee6b : Constant  Value=897.597901025655
  Product_11087 : Product
  Product_4dbb5 : Product
  Product_9a2cc : Product
  Product_dda24 : Product
  Subtract_8a359 : Sum  Inputs=+-
  Subtract_953b9 : Sum  Inputs=+-
  Blockout_d_iq_line_27_29_c732b : Outport
  wires:
  Constant_-376.991118430775_e3c81/1 -> Product_11087/1
  Constant_197.471538225644_20461/1 -> Product_4dbb5/1
  Product_4dbb5/1 -> Subtract_8a359/2
  State_id_line_27_29_86314/1 -> Product_11087/2
  State_iq_line_27_29_e2b12/1 -> Product_4dbb5/2
  Product_dda24/1 -> Add_01c7b/2
  Constant_897.597901025655_7ee6b/1 -> Product_dda24/1
  Product_11087/1 -> Subtract_8a359/1
  State_vq_bus_27_cc3b8/1 -> Product_dda24/2
  Subtract_8a359/1 -> Add_01c7b/1
  Product_9a2cc/1 -> Subtract_953b9/2
  Constant_897.597901025655_51739/1 -> Product_9a2cc/1
  Add_01c7b/1 -> Subtract_953b9/1
  State_vq_bus_29_394c9/1 -> Product_9a2cc/2
  Subtract_953b9/1 -> Blockout_d_iq_line_27_29_c732b/1

== system IEEE30_case/AC_1/d_iq_line_27_30_block ==
  note: d_iq_line_27_30 in IEEE30_case
      | $628.318530717959\,\mathrm{vq}_{\mathrm{bus},27}-201.061929829747\,\mathrm{iq}_{\mathrm{line},27,30}-376.991118430775\,\mathrm{id}_{\mathrm{line},27,30}-628.318530717959\,\mathrm{vq}_{\mathrm{bus},30}$
      | Automatically generated on 2025-11-01 18:42:23 .
  State_id_line_27_30_d18cd : Inport
  State_iq_line_27_30_e9a72 : Inport  Port=2
  State_vq_bus_27_cb66b : Inport  Port=3
  State_vq_bus_30_735a2 : Inport  Port=4
  Add_49de3 : Sum
  Constant_-376.991118430775_9f105 : Constant  Value=-376.991118430775
  Constant_201.061929829747_1a814 : Constant  Value=201.061929829747
  Constant_628.318530717959_0595b : Constant  Value=628.318530717959
  Constant_628.318530717959_57c1b : Constant  Value=628.318530717959
  Product_27e9a : Product
  Product_adc8e : Product
  Product_b0334 : Product
  Product_e8336 : Product
  Subtract_98447 : Sum  Inputs=+-
  Subtract_f359c : Sum  Inputs=+-
  Blockout_d_iq_line_27_30_4beb9 : Outport
  wires:
  Product_b0334/1 -> Subtract_98447/1
  Constant_-376.991118430775_9f105/1 -> Product_b0334/1
  Subtract_f359c/1 -> Blockout_d_iq_line_27_30_4beb9/1
  State_id_line_27_30_d18cd/1 -> Product_b0334/2
  Constant_201.061929829747_1a814/1 -> Product_e8336/1
  Product_e8336/1 -> Subtract_98447/2
  State_iq_line_27_30_e9a72/1 -> Product_e8336/2
  Subtract_98447/1 -> Add_49de3/1
  Constant_628.318530717959_0595b/1 -> Product_27e9a/1
  State_vq_bus_27_cb66b/1 -> Product_27e9a/2
  Product_27e9a/1 -> Add_49de3/2
  Product_adc8e/1 -> Subtract_f359c/2
  Constant_628.318530717959_57c1b/1 -> Product_adc8e/1
  State_vq_bus_30_735a2/1 -> Product_adc8e/2
  Add_49de3/1 -> Subtract_f359c/1

== system IEEE30_case/AC_1/d_iq_line_28_27_block ==
  note: d_iq_line_28_27 in IEEE30_case
      | $942.477796076938\,\mathrm{vq}_{\mathrm{bus},28}-942.477796076938\,\mathrm{vq}_{\mathrm{bus},27}-376.991118430775\,\mathrm{id}_{\mathrm{line},28,27}$
      | Automatically generated on 2025-11-01 18:42:19 .
  State_id_line_28_27_3a5d8 : Inport
  State_vq_bus_27_b0dc4 : Inport  Port=2
  State_vq_bus_28_55731 : Inport  Port=3
  Add_d99cf : Sum
  Constant_-376.991118430775_69e07 : Constant  Value=-376.991118430775
  Constant_942.477796076938_60c4b : Constant  Value=942.477796076938
  Constant_942.477796076938_81c09 : Constant  Value=942.477796076938
  Product_49ce4 : Product
  Product_6b0a6 : Product
  Product_d5be0 : Product
  Subtract_b567c : Sum  Inputs=+-
  Blockout_d_iq_line_28_27_81b11 : Outport
  wires:
  Constant_-376.991118430775_69e07/1 -> Product_d5be0/1
  Constant_942.477796076938_81c09/1 -> Product_6b0a6/1
  Product_6b0a6/1 -> Subtract_b567c/2
  State_id_line_28_27_3a5d8/1 -> Product_d5be0/2
  State_vq_bus_27_b0dc4/1 -> Product_6b0a6/2
  Product_d5be0/1 -> Subtract_b567c/1
  Product_49ce4/1 -> Add_d99cf/2
  Constant_942.477796076938_60c4b/1 -> Product_49ce4/1
  State_vq_bus_28_55731/1 -> Product_49ce4/2
  Subtract_b567c/1 -> Add_d99cf/1
  Add_d99cf/1 -> Blockout_d_iq_line_28_27_81b11/1

== system IEEE30_case/AC_1/d_iq_line_29_30_block ==
  note: d_iq_line_29_30 in IEEE30_case
      | $837.758040957278\,\mathrm{vq}_{\mathrm{bus},29}-201.061929829747\,\mathrm{iq}_{\mathrm{line},29,30}-376.991118430775\,\mathrm{id}_{\mathrm{line},29,30}-837.758040957278\,\mathrm{vq}_{\mathrm{bus},30}$
      | Automatically generated on 2025-11-01 18:42:26 .
  State_id_line_29_30_717f3 : Inport
  State_iq_line_29_30_5dcc0 : Inport  Port=2
  State_vq_bus_29_3e7b3 : Inport  Port=3
  State_vq_bus_30_6aab5 : Inport  Port=4
  Add_38d0d : Sum
  Constant_-376.991118430775_58bdb : Constant  Value=-376.991118430775
  Constant_201.061929829747_813ad : Constant  Value=201.061929829747
  Constant_837.758040957278_16bd2 : Constant  Value=837.758040957278
  Constant_837.758040957278_27438 : Constant  Value=837.758040957278
  Product_b3d73 : Product
  Product_b8a27 : Product
  Product_cccc9 : Product
  Product_f6a99 : Product
  Subtract_6af12 : Sum  Inputs=+-
  Subtract_9cebf : Sum  Inputs=+-
  Blockout_d_iq_line_29_30_05166 : Outport
  wires:
  Constant_-376.991118430775_58bdb/1 -> Product_f6a99/1
  Constant_837.758040957278_16bd2/1 -> Product_b8a27/1
  Product_f6a99/1 -> Subtract_9cebf/1
  State_id_line_29_30_717f3/1 -> Product_f6a99/2
  Constant_201.061929829747_813ad/1 -> Product_cccc9/1
  Product_cccc9/1 -> Subtract_9cebf/2
  Product_b3d73/1 -> Add_38d0d/2
  Constant_837.758040957278_27438/1 -> Product_b3d73/1
  State_iq_line_29_30_5dcc0/1 -> Product_cccc9/2
  State_vq_bus_29_3e7b3/1 -> Product_b3d73/2
  Subtract_9cebf/1 -> Add_38d0d/1
  State_vq_bus_30_6aab5/1 -> Product_b8a27/2
  Add_38d0d/1 -> Subtract_6af12/1
  Product_b8a27/1 -> Subtract_6af12/2
  Subtract_6af12/1 -> Blockout_d_iq_line_29_30_05166/1

== system IEEE30_case/AC_1/d_iq_line_2_4_block ==
  note: d_iq_line_2_4 in IEEE30_case
      | $2217.59481429868\,\mathrm{vq}_{\mathrm{bus},2}-133.055688857921\,\mathrm{iq}_{\mathrm{line},2,4}-376.991118430775\,\mathrm{id}_{\mathrm{line},2,4}-2217.59481429868\,\mathrm{vq}_{\mathrm{bus},4}$
      | Automatically generated on 2025-11-01 18:41:02 .
  State_id_line_2_4_7fbc5 : Inport
  State_iq_line_2_4_b638e : Inport  Port=2
  State_vq_bus_2_08b2a : Inport  Port=3
  State_vq_bus_4_bf96b : Inport  Port=4
  Add_9c8ee : Sum
  Constant_-376.991118430775_825b8 : Constant  Value=-376.991118430775
  Constant_133.055688857921_0be5f : Constant  Value=133.055688857921
  Constant_2217.59481429868_03ef9 : Constant  Value=2217.59481429868
  Constant_2217.59481429868_4692e : Constant  Value=2217.59481429868
  Product_2f0b3 : Product
  Product_3cb4b : Product
  Product_61fd1 : Product
  Product_7c15d : Product
  Subtract_8c8cb : Sum  Inputs=+-
  Subtract_eaf1f : Sum  Inputs=+-
  Blockout_d_iq_line_2_4_be6c7 : Outport
  wires:
  State_vq_bus_2_08b2a/1 -> Product_3cb4b/2
  Constant_-376.991118430775_825b8/1 -> Product_2f0b3/1
  Constant_2217.59481429868_4692e/1 -> Product_3cb4b/1
  State_id_line_2_4_7fbc5/1 -> Product_2f0b3/2
  Constant_133.055688857921_0be5f/1 -> Product_7c15d/1
  Product_7c15d/1 -> Subtract_8c8cb/2
  Product_2f0b3/1 -> Subtract_8c8cb/1
  State_iq_line_2_4_b638e/1 -> Product_7c15d/2
  Subtract_8c8cb/1 -> Add_9c8ee/1
  Product_3cb4b/1 -> Add_9c8ee/2
  Product_61fd1/1 -> Subtract_eaf1f/2
  Constant_2217.59481429868_03ef9/1 -> Product_61fd1/1
  State_vq_bus_4_bf96b/1 -> Product_61fd1/2
  Add_9c8ee/1 -> Subtract_eaf1f/1
  Subtract_eaf1f/1 -> Blockout_d_iq_line_2_4_be6c7/1
